simulink model "ss_kalmf_Observer"  (R2022b)
settings: Solver=FixedStepDiscrete  StartTime=0.0  StopTime=10.0  RelTol=1e-3
settings Model: Creator=hp_desktop  LastModifiedBy=hp_desktop
settings DataIOCC: SaveOutput=off  SaveTime=off

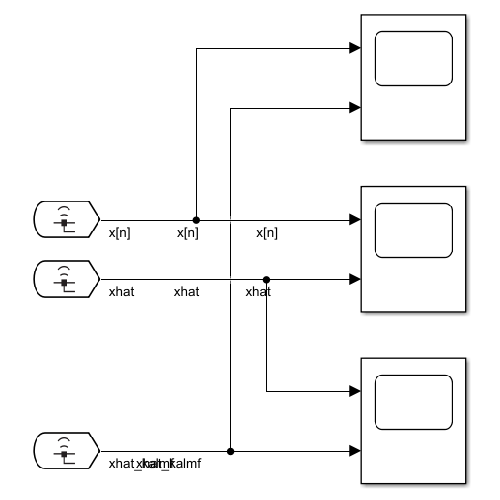
[thumbnail: Simulink's stored preview of the top-level diagram]
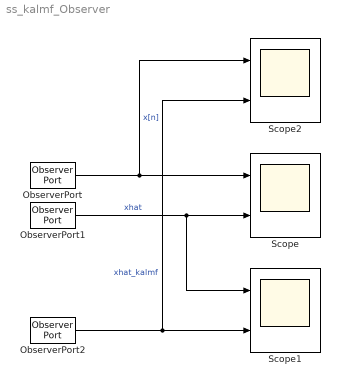
== system ss_kalmf_Observer ==
  ObserverPort : ObserverPort
  ObserverPort1 : ObserverPort
  ObserverPort2 : ObserverPort
  Scope : Scope  NumInputPorts=2
  Scope1 : Scope  NumInputPorts=2
  Scope2 : Scope  NumInputPorts=2
  wires:
  ObserverPort/1 -> Scope2/1, Scope/1  "x[n]"
  ObserverPort1/1 -> Scope1/1, Scope/2  "xhat"
  ObserverPort2/1 -> Scope2/2, Scope1/2  "xhat_kalmf"
